simulink model "loopshaping"  (R2015a)
settings: Solver=ode3  StartTime=0.0  StopTime=10.0  FixedStep=1/200  RelTol=1e-3
libraries: PoliArd x5, simulink x3
settings Model: ExtModeTrigDuration=2  Creator=GSavaia  LastModifiedBy=GSavaia
settings OptimizationCC: OptimizeModelRefInitCode=on  LifeSpan=1
settings DebuggingCC: UnderspecifiedInitializationDetection=Classic  MergeDetectMultiDrivingBlocksExec=none
settings HardwareCC: ProdLargestAtomicInteger=Long  ProdLargestAtomicFloat=Double  ProdEndianess=LittleEndian  ProdHWDeviceType=ARM Compatible->ARM Cortex
settings RTWCC: SystemTargetFile=realtime.tlc  GenerateMakefile=off  TemplateMakefile=realtime.tmf  Description=Run on Target Hardware  RTWVerbose=off
settings ERTTargetCC: CombineOutputUpdateFcns=off  ExtModeTransport=3  ExtModeMexFile=ext_serial_win32_comm_rtt  ExtModeMexArgs=0 1 9600  ERTSrcFileBannerTemplate=realtime_code_template.cgt  ERTHdrFileBannerTemplate=realtime_code_template.cgt  ERTDataSrcFileTemplate=realtime_code_template.cgt  ERTDataHdrFileTemplate=realtime_code_template.cgt  ERTCustomFileTemplate=realtime_file_process.tlc

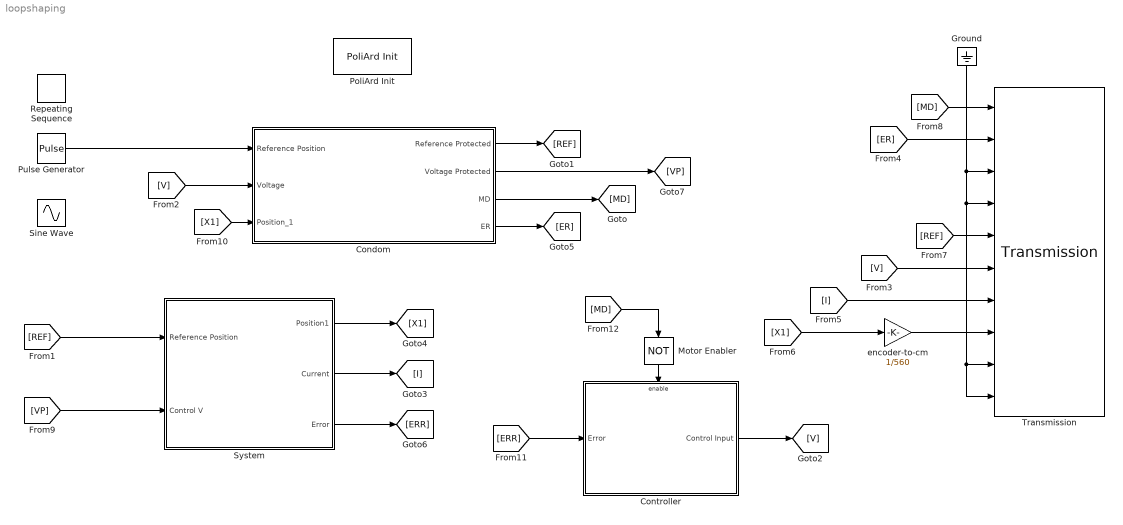
== system loopshaping ==
  Condom : Subsystem
  Controller : Subsystem
  Ground : Ground
  Motor Enabler : Logic  Operator=NOT  AllPortsSameDT=off  OutDataTypeStr=boolean
  PoliArd Init : PoliArd/PoliArd Init
  Pulse Generator : DiscretePulseGenerator  PulseType=Time based  Period=10  PulseWidth=50
  Repeating Sequence : simulink/Sources/Repeating Sequence  rep_seq_t=[0 5]  rep_seq_y=[0 1]
  Sine Wave : Sin  Amplitude=0.5  Bias=0.5  Frequency=2*pi  SampleTime=0
  "System " : Subsystem
  Transmission : PoliArd/Transmission  sample_freq=200  sig_to_send=6
  encoder-to-cm : Gain  Gain=1/560
  wires:
  Condom/1(Reference Protected) -> [REF]
  [REF] -> "System "/1(Reference Position)
  "System "/2(Current) -> [I]
  [V] -> Condom/2(Voltage)
  [V] -> Transmission/6
  [I] -> Transmission/7
  "System "/1(Position1) -> [X1]
  [X1] -> encoder-to-cm/1
  [REF] -> Transmission/5
  [MD] -> Transmission/1
  [VP] -> "System "/2(Control V)
  [X1] -> Condom/3(Position_1)
  encoder-to-cm/1 -> Transmission/8
  Controller/1(Control Input) -> [V]
  "System "/3(Error) -> [ERR]
  [ERR] -> Controller/1(Error)
  Condom/2("Voltage Protected ") -> [VP]
  Condom/3(MD) -> [MD]
  Condom/4(ER) -> [ER]
  Ground/1 -> Transmission/9, Transmission/10, Transmission/4, Transmission/3
  Pulse Generator/1 -> Condom/1(Reference Position)
  [ER] -> Transmission/2
  [MD] -> Motor Enabler/1
  Motor Enabler/1 -> Controller/Enable

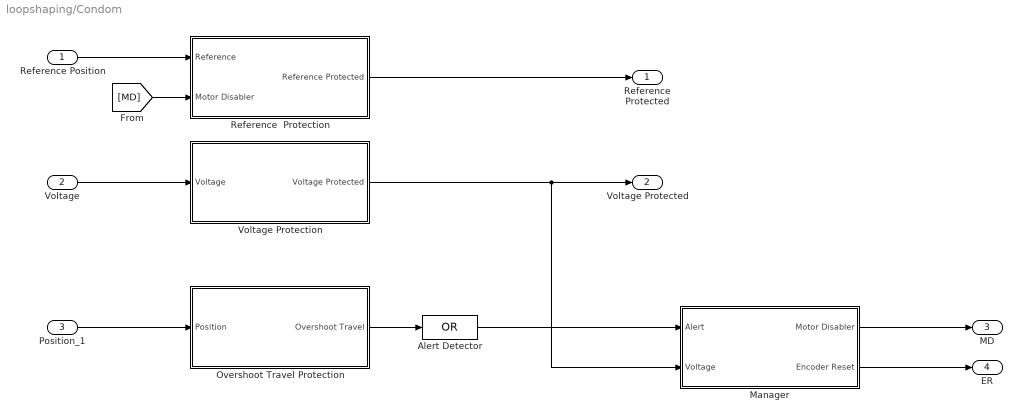
== system loopshaping/Condom ==
  Reference Position : Inport
  Voltage : Inport  Port=2
  Position_1 : Inport  Port=3
  Alert Detector : Logic  Operator=OR  Inputs=1  AllPortsSameDT=off  OutDataTypeStr=boolean
  Manager : Subsystem
  Overshoot Travel Protection : Subsystem
  Reference  Protection : Subsystem
  Voltage Protection : Subsystem
  Reference Protected : Outport
  "Voltage Protected " : Outport  Port=2
  MD : Outport  Port=3
  ER : Outport  Port=4
  wires:
  Reference Position/1 -> Reference  Protection/1("Reference ")
  Position_1/1 -> Overshoot Travel Protection/1("Position ")
  Overshoot Travel Protection/1(Overshoot Travel) -> Alert Detector/1
  Voltage/1 -> Voltage Protection/1("Voltage ")
  Voltage Protection/1(Voltage Protected) -> Manager/2(Voltage), "Voltage Protected "/1
  Reference  Protection/1(Reference Protected) -> Reference Protected/1
  Alert Detector/1 -> Manager/1(Alert)
  Manager/2(Encoder Reset) -> ER/1
  Manager/1(Motor Disabler) -> MD/1
  [MD] -> Reference  Protection/2(Motor Disabler)

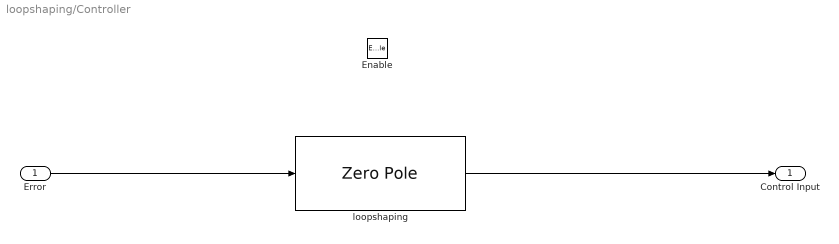
== system loopshaping/Controller ==
  Error : Inport
  Enable : EnablePort  StatesWhenEnabling=reset
  loopshaping : ZeroPole  Zeros=[-3.5+22i, -3.5-22i]  Poles=[0, -100]  Gain=-0.005
  Control Input : Outport
  wires:
  Error/1 -> loopshaping/1
  loopshaping/1 -> Control Input/1

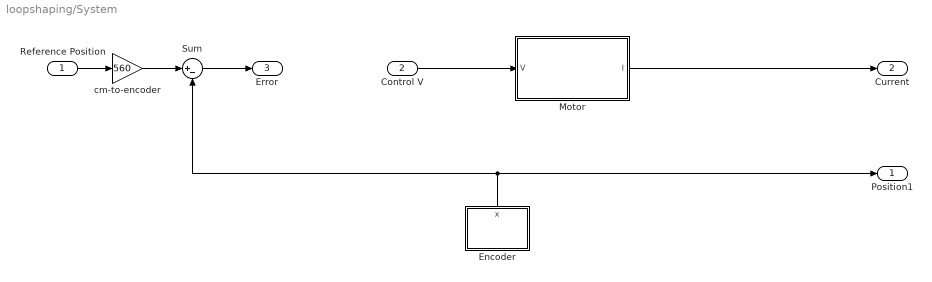
== system loopshaping/System  ==
  Reference Position : Inport
  Control V : Inport  Port=2
  "Encoder " : Subsystem
  Motor : Subsystem
  Sum : Sum  Inputs=|+-
  cm-to-encoder : Gain  Gain=560
  Position1 : Outport
  Current : Outport  Port=2
  Error : Outport  Port=3
  wires:
  "Encoder "/1(x) -> Position1/1, Sum/2
  cm-to-encoder/1 -> Sum/1
  Motor/1(I) -> Current/1
  Sum/1 -> Error/1
  Reference Position/1 -> cm-to-encoder/1
  Control V/1 -> Motor/1(V)

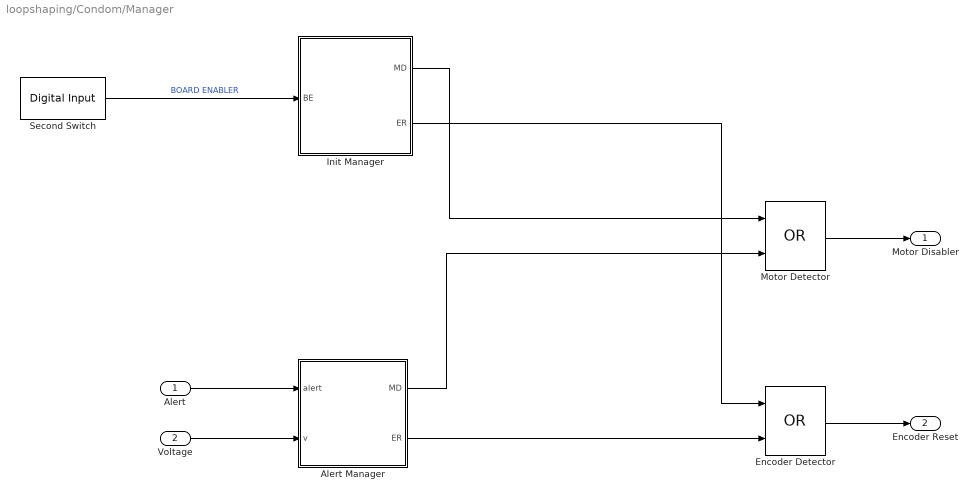
== system loopshaping/Condom/Manager ==
  Alert : Inport
  Voltage : Inport  Port=2
  Alert Manager : Stateflow chart  TreatAsAtomicUnit=on
  Encoder Detector : Logic  Operator=OR  AllPortsSameDT=off  OutDataTypeStr=boolean
  Init Manager : Stateflow chart  TreatAsAtomicUnit=on
  Motor Detector : Logic  Operator=OR  AllPortsSameDT=off  OutDataTypeStr=boolean
  Second Switch : PoliArd/Digital Input  DI_pin=2  DIsample=1/200
  Motor Disabler : Outport
  Encoder Reset : Outport  Port=2
  wires:
  Second Switch/1 -> Init Manager/1(BE)  "BOARD ENABLER"
  Motor Detector/1 -> Motor Disabler/1
  Encoder Detector/1 -> Encoder Reset/1
  Init Manager/1(MD) -> Motor Detector/1
  Alert Manager/1(MD) -> Motor Detector/2
  Init Manager/2(ER) -> Encoder Detector/1
  Alert Manager/2(ER) -> Encoder Detector/2
  Alert/1 -> Alert Manager/1(alert)
  Voltage/1 -> Alert Manager/2(v)

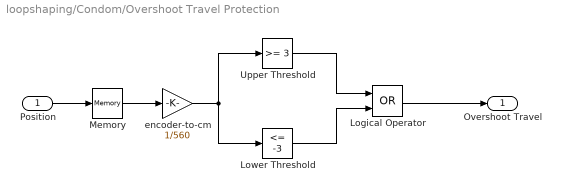
== system loopshaping/Condom/Overshoot Travel Protection ==
  "Position " : Inport
  Logical Operator : Logic  Operator=OR  AllPortsSameDT=off  OutDataTypeStr=boolean
  Lower Threshold : simulink/Logic and Bit Operations/Compare To Constant  relop=<=  const=-3  OutDataTypeStr=boolean
  Memory : Memory
  Upper Threshold : simulink/Logic and Bit Operations/Compare To Constant  relop=>=  const=3  OutDataTypeStr=boolean
  encoder-to-cm : Gain  Gain=1/560
  Overshoot Travel : Outport
  wires:
  Logical Operator/1 -> Overshoot Travel/1
  Lower Threshold/1 -> Logical Operator/2
  Upper Threshold/1 -> Logical Operator/1
  "Position "/1 -> Memory/1
  encoder-to-cm/1 -> Lower Threshold/1, Upper Threshold/1
  Memory/1 -> encoder-to-cm/1

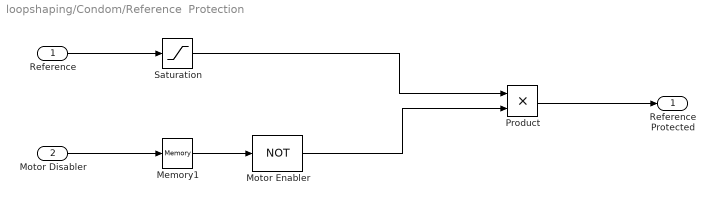
== system loopshaping/Condom/Reference  Protection ==
  "Reference " : Inport
  Motor Disabler : Inport  Port=2
  Memory1 : Memory
  Motor Enabler : Logic  Operator=NOT  Inputs=1  AllPortsSameDT=off  OutDataTypeStr=boolean
  Product : Product
  Saturation : Saturate  UpperLimit=3  LowerLimit=-3
  Reference Protected : Outport
  wires:
  "Reference "/1 -> Saturation/1
  Saturation/1 -> Product/1
  Motor Enabler/1 -> Product/2
  Memory1/1 -> Motor Enabler/1
  Product/1 -> Reference Protected/1
  Motor Disabler/1 -> Memory1/1

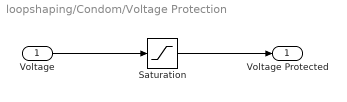
== system loopshaping/Condom/Voltage Protection ==
  "Voltage " : Inport
  Saturation : Saturate  UpperLimit=5  LowerLimit=-5
  Voltage Protected : Outport
  wires:
  Saturation/1 -> Voltage Protected/1
  "Voltage "/1 -> Saturation/1

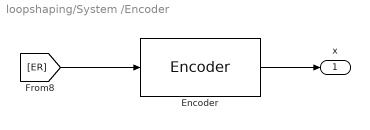
== system loopshaping/System /Encoder  ==
  Encoder : PoliArd/Encoder  EncoderID=1  dt_enc=1/200
  x : Outport
  wires:
  Encoder/1 -> x/1
  [ER] -> Encoder/1

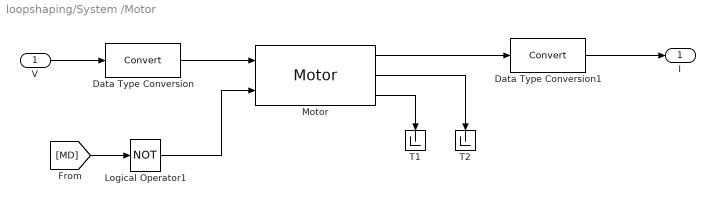
== system loopshaping/System /Motor ==
  V : Inport
  Data Type Conversion : DataTypeConversion
  Data Type Conversion1 : DataTypeConversion
  Logical Operator1 : Logic  Operator=NOT  AllPortsSameDT=off  OutDataTypeStr=boolean
  Motor : PoliArd/Motor  MotorID=2  DC_bus_mask=12  dt_mot=1/200
  T1 : Terminator
  T2 : Terminator
  I : Outport
  wires:
  Data Type Conversion/1 -> Motor/1
  V/1 -> Data Type Conversion/1
  Motor/3 -> T1/1
  Motor/2 -> T2/1
  Motor/1 -> Data Type Conversion1/1
  Data Type Conversion1/1 -> I/1
  Logical Operator1/1 -> Motor/2
  [MD] -> Logical Operator1/1

== stateflow chart loopshaping/Condom/Manager/Init Manager ==
  state STOP
    entry:
    MD = 1;
    ER = 1;
  state OPERATIVE
    entry:
    MD = 0;
    ER = 0;
  state INIT
    entry:
    MD = 1;
    ER  = 1;
  (default) -> STOP
  OPERATIVE -> STOP : [BE==0]
  STOP -> INIT : [BE==1]
  INIT -> OPERATIVE : after(3, sec)
  data: MD output; ER output; BE input

== stateflow chart loopshaping/Condom/Manager/Alert Manager ==
  state OK
    entry:
    MD=0;
    ER=0;
  state ALERT
    entry:
    MD=1;
    ER=1;
  (default) -> OK
  OK -> ALERT : [alert==1]
  ALERT -> OK : [abs(v)<0.3]
  data: alert input; v input; MD output; ER output
